simulink subsystem "nco"  (R2021a)
settings: Solver=VariableStepAuto  StartTime=0.0  StopTime=10.0  RelTol=1e-3
libraries: xbsIndex_r4 x7
settings Model: Creator=casper  LastModifiedBy=casper

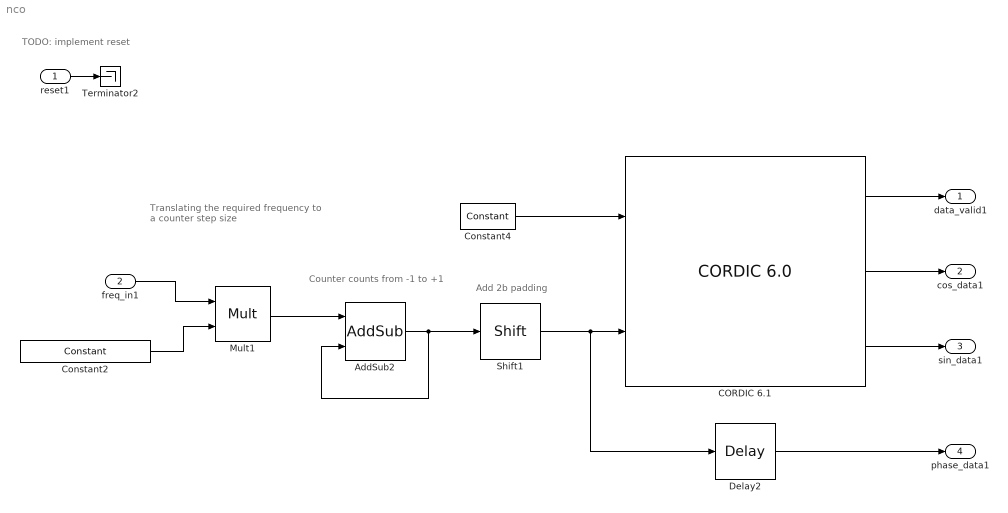
== system nco ==
  note: TODO: implement reset
  note: Add 2b padding
  note: Counter counts from -1 to +1
  note: Translating the required frequency
      | to a counter step size
  reset1 : Inport
  freq_in1 : Inport  Port=2
  AddSub2 : xbsIndex_r4/AddSub  mode=Addition  use_carryin=off  use_carryout=off  en=off  latency=1  precision=User Defined  arith_type="Signed  (2's comp)"  n_bits=36  bin_pt=35  quantization="Round  (unbiased: +/- Inf)"  overflow=Wrap  use_behavioral_HDL=off  hw_selection=Fabric  pipelined=off  dbl_ovrd=off  block_type=addsub
  CORDIC 6.1 : xbsIndex_r4/CORDIC 6.0   functional_selection=Sin_and_Cos  architectural_configuration=Parallel  pipelining_mode=Optimal  data_format=SignedFraction  phase_format=Scaled_Radians  input_width=32  output_width=14  round_mode=Truncate  iterations=0  precision=0  compensation_scaling=No_Scale_Compensation  coarse_rotation=on  aclken=off  aresetn=off  out_tready=off  cartesian_has_tuser=off  cartesian_has_tlast=off  cartesian_tuser_width=1  phase_has_tuser=off  phase_has_tlast=off  phase_tuser_width=1  out_tlast_behv=Null  flow_control=NonBlocking  optimize_goal=Resources  trim_axipin_name=on  simulation_type=hybrid_sim  simulation_model=sysgen:cordic_v6_0  data_path_portlist={'s_axis_cartesian_tdata_imag', 's_axis_cartesian_tdata_real', 's_axis_phase_tdata_phase', 'm_axis_dout_tdata_imag', 'm_axis_dout_tdata_real', 'm_axis_dout_tdata_phase','m_axis_dout_tdata'}  ip_name=CORDIC  ip_version=6.0  dsptool_ready=true  ipcore_usecache=true  ipcore_useipmodelcache=true  wrapper_available=true  port_translation_map={ 'aclken' => 'en', 'aresetn' => 'rst' }  block_type=cordic_v6_0
      settings: infoedit=CORDIC 6.0
  Constant2 : xbsIndex_r4/Constant  const=2/125000000  gui_display_data_type=Fixed-point  arith_type=Unsigned  n_bits=64  bin_pt=64  preci_type=Single  exp_width=8  frac_width=24  explicit_period=on  period=1  equ=P=C  opselect=C  inp2=PCIN>>17  opr=+  inp1=P  carry=CIN  dbl_ovrd=off  block_type=constant
  Constant4 : xbsIndex_r4/Constant  const=1.0  gui_display_data_type=Boolean  arith_type=Boolean  n_bits=16  bin_pt=14  preci_type=Single  exp_width=8  frac_width=24  explicit_period=on  period=1  equ=P=C  opselect=C  inp2=PCIN>>17  opr=+  inp1=P  carry=CIN  dbl_ovrd=off  block_type=constant
  Delay2 : xbsIndex_r4/Delay  rst=off  infoeditControl=Selection of Reset will increase slice count due to use of real FFs and instead of SRLs  en=off  latency=17  reg_retiming=off  dbl_ovrd=off  block_type=delay
  Mult1 : xbsIndex_r4/Mult  precision=Full  arith_type="Signed  (2's comp)"  n_bits=16  bin_pt=14  quantization=Truncate  overflow=Wrap  en=off  latency=3  use_behavioral_HDL=off  opt=Speed  use_embedded=on  optimum_pipeline=off  pipeline=on  dbl_ovrd=off  use_rpm=on  placement_style=Triangular  block_type=mult
  Shift1 : xbsIndex_r4/Shift  shift_dir=Right  shift_bits=0  en=off  latency=1  precision=User Defined  arith_type="Signed  (2's comp)"  n_bits=38  bin_pt=35  quantization=Truncate  overflow=Wrap  dbl_ovrd=off  block_type=shift
  Terminator2 : Terminator
  data_valid1 : Outport
  cos_data1 : Outport  Port=2
  sin_data1 : Outport  Port=3
  phase_data1 : Outport  Port=4
  wires:
  CORDIC 6.1/3 -> sin_data1/1
  Shift1/1 -> CORDIC 6.1/2, Delay2/1
  AddSub2/1 -> Shift1/1, AddSub2/2
  CORDIC 6.1/2 -> cos_data1/1
  reset1/1 -> Terminator2/1
  Constant4/1 -> CORDIC 6.1/1
  Delay2/1 -> phase_data1/1
  Mult1/1 -> AddSub2/1
  Constant2/1 -> Mult1/2
  CORDIC 6.1/1 -> data_valid1/1
  freq_in1/1 -> Mult1/1
